simulink model "p5"  (Simulink 7.5)
settings: Solver=ode23t  StartTime=0.0  StopTime=1.0  MaxStep=1e-6  RelTol=1e-3
libraries: powerlib x7
settings Model: Creator=dell 15  LastModifiedBy=dell 15

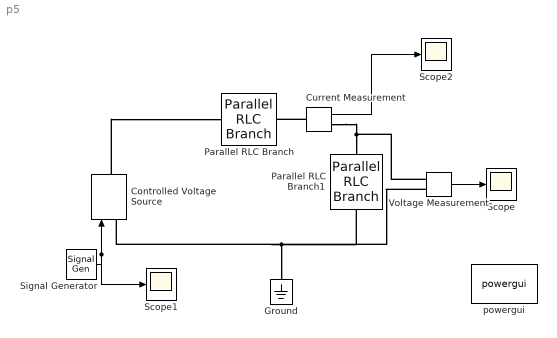
== system p5 ==
  Controlled Voltage Source : powerlib/Electrical Sources/Controlled Voltage Source  DialogController=POWERSYS.PowerSysDialog  SystemSampleTime=-1  Initialize=on  Source_Type=AC  Amplitude=0  Phase=0  Frequency=0  Measurements=None
  Current Measurement : powerlib/Measurements/Current Measurement  DialogController=POWERSYS.PowerSysDialog  SystemSampleTime=-1  PhasorSimulation=off  OutputType=Complex  PSBequivalent=0
  Ground : powerlib/Elements/Ground  DialogController=POWERSYS.PowerSysDialog  PhysicalDomain=powersysdomain  SubClassName=unknown  LeftPortType=p1  RightPortType=p1  LConnTagsString=a
  Parallel RLC Branch : powerlib/Elements/Parallel RLC Branch  DialogController=POWERSYS.PowerSysDialog  PhysicalDomain=powersysdomain  SubClassName=unknown  LeftPortType=p1  RightPortType=p1  LConnTagsString=a  RConnTagsString=__new0  BranchType=R  Resistance=1000  Inductance=1e-3  SetiL0=off  InitialCurrent=0  Capacitance=1e-6  Setx0=off  InitialVoltage=0  Measurements=None
  Parallel RLC Branch1 : powerlib/Elements/Parallel RLC Branch  DialogController=POWERSYS.PowerSysDialog  PhysicalDomain=powersysdomain  SubClassName=unknown  LeftPortType=p1  RightPortType=p1  LConnTagsString=a  RConnTagsString=__new0  BranchType=C  Resistance=1  Inductance=1e-3  SetiL0=off  InitialCurrent=0  Capacitance=.2e-6  Setx0=off  InitialVoltage=0  Measurements=None
  Scope : Scope
      settings: YMin=-5e-005  YMax=5e-005
  Scope1 : Scope
      settings: YMin=-5.5e-005  YMax=5.5e-005
  Scope2 : Scope
      settings: SaveName=ScopeData2
  Signal Generator : SignalGenerator  Amplitude=20  Frequency=50
  Voltage Measurement : powerlib/Measurements/Voltage Measurement  DialogController=POWERSYS.PowerSysDialog  SystemSampleTime=-1  PhasorSimulation=off  OutputType=Complex  PSBequivalent=0
  powergui : powerlib/powergui  Priority=1  SystemSampleTime=-1  SimulationMode=Continuous  SampleTime=50e-6  frequency=60  SPID=off  DisableSnubberDevices=off  DisableRonSwitches=off  DisableVfSwitches=off  SwTol=0  Interpol=off  frequencyindice=0  echomessages=off  HookPort=off  DisplayEquations=off  FunctionMessages=off  EnableUseOfTLC=off  x0status=blocks  RestoreLinks=warning  ResistiveCurrentMeasurement=off  Ylog=off  Xlog=on  ShowGrid=off  save=off  variable=ZData  ZoomFFT=off  StartTime=0.0  cycles=1  DisplayStyle=1  FreqAxis=off  MaxFrequency=1000  frequencyindicesteady=1  display=off  methode=off
  wires:
  Voltage Measurement/1 -> Scope/1
  Signal Generator/1 -> Controlled Voltage Source/1, Scope1/1
  Current Measurement/1 -> Scope2/1
  connections:
  Controlled Voltage Source/RConn1 -- Parallel RLC Branch/LConn1
  Voltage Measurement/LConn1 -- Parallel RLC Branch1/LConn1 -- Current Measurement/RConn1
  Voltage Measurement/LConn2 -- Parallel RLC Branch1/RConn1 -- Controlled Voltage Source/LConn1 -- Ground/LConn1
  Current Measurement/LConn1 -- Parallel RLC Branch/RConn1
